simulink model "rugos_rendszer_new"  (R2019b)
settings: Solver=ode23  StartTime=0  StopTime=5  MaxStep=0.1  RelTol=1e-3  AbsTol=1e-6
PostLoadFcn:
  | crtanim2([],[],[],0,1);
model workspace (MAT data in the model file):
  K = [3.08189689488 2.48269889228 0.0803807652926 3.18658131281]
  ae = [0  1  -31.4507297013  0; -1  0  44.8536687603  0; 0  0  -46.6599405981  1; 1  0  -89.5750283103  0]
  be = [0  31.4507297013; 1  -43.8536687603; 0  46.6599405981; 0  88.5750283103]
  ce = [1  0  0  0; 0  1  0  0; 0  0  1  0; 0  0  0  1]
  de = [0  0; 0  0; 0  0; 0  0]
  ka = 1
  m1 = 1
  m2 = 1
  xBx1 = [0; 0; -2; -2; 0]
  xBx2 = [0; 2; 2; 0; 0]
  xSpr = [0; 0.4; 0.8; 1.6; 2.4; 3.2; 3.6; 4]
values from neighbouring files (symbols this model uses):
  k = 2    [Untitled.m]
  Kfb = -inv(R)*B'*P    [Untitled.m]
  Kff = -inv(R)*B'*((A-B*inv(R)*B'*P)')^(-1)*C'*Q    [Untitled.m]
  M1 = 50    [Untitled.m]
  M2 = 10    [Untitled.m]
Description:
  | Double Spring Mass System
  | 
  | This example shows how to model a double spring-mass-damper system with a periodically
  | varying forcing function.  Associated with the example is an animation function
  | that will automatically open a figure window and display to it. In this system,
  | the only sensor is attached to the mass on the left, and the actuator is
  | attached to the mass on the left. State estimation and LQR control are used.
settings Model: ExtModeAutoUpdateStatusClock=off  Creator=The MathWorks, Inc.  LastModifiedBy=patti
settings SolverCC: AutoScaleAbsTol=off
settings DataIOCC: ExternalInput=[]  InitialState=[]  SaveFormat=Array  SaveOutput=off  SaveTime=off  ReturnWorkspaceOutputs=off
settings OptimizationCC: BlockReduction=off  BooleanDataType=off  InitFltsAndDblsToZero=on  LifeSpan=inf  BufferReusableBoundary=off
settings DebuggingCC: SaveWithParameterizedLinksMsg=none  UnderspecifiedInitializationDetection=Classic  MergeDetectMultiDrivingBlocksExec=none  SignalResolutionControl=TryResolveAllWithWarning  MultiTaskDSMMsg=warning  MultiTaskCondExecSysMsg=none  FcnCallInpInsideContextMsg=warning  BusObjectLabelMismatch=none  SFUnexpectedBacktrackingDiag=warning  SFNoUnconditionalDefaultTransitionDiag=warning  SFExecutionAtInitializationDiag=none  ArithmeticOperatorsInVariantConditions=warning
settings HardwareCC: ProdBitPerPointer=32  ProdBitPerSizeT=32  ProdBitPerPtrDiffT=32  ProdLargestAtomicFloat=None  ProdIntDivRoundTo=Undefined  ProdEndianess=Unspecified  ProdWordSize=32  ProdHWDeviceType=32-bit Generic  TargetUnknown=on
settings ModelReferenceCC: PropagateSignalLabelsOutOfModel=off
settings SFSimCC: SimUseLocalCustomCode=off  CustomCodeUndefinedFunction=UseInterfaceOnly
settings RTWCC: Description=Generic Real-Time Target  RTWUseLocalCustomCode=off
settings CodeAppCC: StateflowObjectComments=on
settings GRTTargetCC: TargetFcnLib=ansi_tfl_tmw.mat  TargetLangStandard=C89/C90 (ANSI)  GeneratePreprocessorConditionals=Disable all  CombineOutputUpdateFcns=off  GRTInterface=on
settings ConfigComp: CovMetricSettings=dw  CovHtmlReporting=on  CovSaveCumulativeToWorkspaceVar=on  CovSaveSingleToWorkspaceVar=on  CovExternalEMLEnable=off

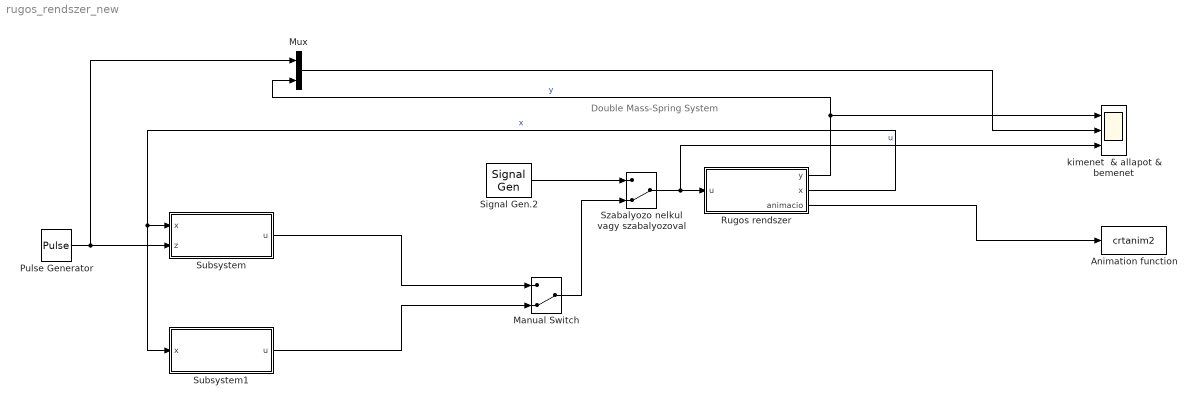
== system rugos_rendszer_new ==
  note: Double Mass-Spring System
  Animation function : S-Function  FunctionName=crtanim2  Parameters=0.1  SFunctionDeploymentMode=off  EnableBusSupport=off
      settings: DeleteFcn=shh = get(0,'ShowHiddenHandles');set(0,'ShowHiddenHandles','on');if ~isempty(findobj('type','figure','name','dblcart1 Animation'));close('dblcart1 Animation'); end;set(0,'ShowHiddenHandles',shh);
  Manual Switch : ManualSwitch  CurrentSetting=0
  Mux : Mux  Inputs=2
  Pulse Generator : DiscretePulseGenerator  PulseType=Time based  Amplitude=5  Period=20  PulseWidth=50
  Rugos rendszer : Subsystem  mask{ka=k, m1=M1, m2=M2}
  Signal Gen.2 : SignalGenerator  WaveForm=square  Amplitude=15  Frequency=0.300000  Units=rad/sec
  Subsystem : Subsystem
  Subsystem1 : Subsystem
  Szabalyozo nelkul vagy szabalyozoval : ManualSwitch  CurrentSetting=0
  kimenet  & allapot & bemenet : Scope  NumInputPorts=3
  wires:
  Signal Gen.2/1 -> Szabalyozo nelkul vagy szabalyozoval/1
  Rugos rendszer/3(animacio) -> Animation function/1
  Szabalyozo nelkul vagy szabalyozoval/1 -> kimenet  & allapot & bemenet/3, Rugos rendszer/1(u)  "u"
  Rugos rendszer/2(x) -> Subsystem1/1("x "), Subsystem/1(x)  "x"
  Manual Switch/1 -> Szabalyozo nelkul vagy szabalyozoval/2
  Subsystem/1("u ") -> Manual Switch/1
  Subsystem1/1("u ") -> Manual Switch/2
  Pulse Generator/1 -> Subsystem/2(z), Mux/1
  Rugos rendszer/1(y) -> kimenet  & allapot & bemenet/1, Mux/2  "y"
  Mux/1 -> kimenet  & allapot & bemenet/2

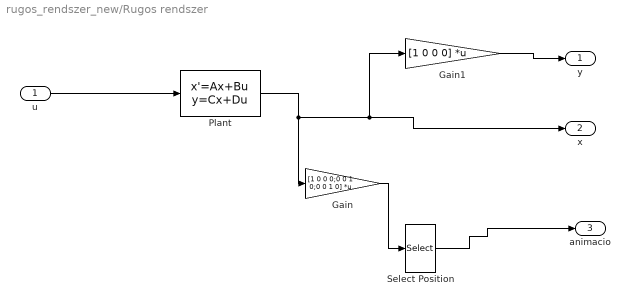
== system rugos_rendszer_new/Rugos rendszer ==
  u : Inport
  Gain : Gain  Gain=[1 0 0 0;0 0 1 0;0 0 1 0]  Multiplication=Matrix(K*u)
  Gain1 : Gain  Gain=[1 0 0 0]  Multiplication=Matrix(K*u)
  Plant : StateSpace  A=[0 1 0 0; -ka/m1 0 ka/m1 0; 0 0 0 1;ka/m2 0 -ka/m2 0]  B=[0; 1; 0; 0]  C=eye(4)  D=zeros(4,1)  InitialCondition=0
  Select Position : Selector  InputPortWidth=3  IndexOptions=Index vector (dialog)  Indices=[1,2]  OutputSizes=1
  y : Outport
  x : Outport  Port=2
  animacio : Outport  Port=3
  wires:
  Select Position/1 -> animacio/1
  u/1 -> Plant/1
  Gain1/1 -> y/1
  Gain/1 -> Select Position/1
  Plant/1 -> Gain1/1, x/1, Gain/1

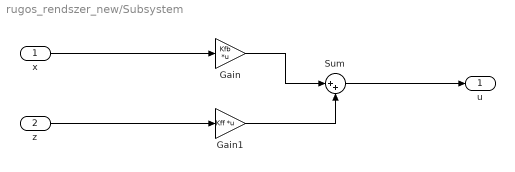
== system rugos_rendszer_new/Subsystem ==
  x : Inport
  z : Inport  Port=2
  Gain : Gain  Gain=Kfb  Multiplication=Matrix(K*u)
  Gain1 : Gain  Gain=Kff  Multiplication=Matrix(K*u)
  Sum : Sum  Inputs=|++
  "u " : Outport
  wires:
  x/1 -> Gain/1
  z/1 -> Gain1/1
  Gain1/1 -> Sum/2
  Gain/1 -> Sum/1
  Sum/1 -> "u "/1

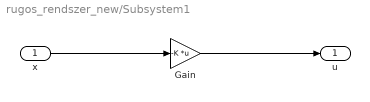
== system rugos_rendszer_new/Subsystem1 ==
  "x " : Inport
  Gain : Gain  Gain=-K  Multiplication=Matrix(K*u)
  "u " : Outport
  wires:
  "x "/1 -> Gain/1
  Gain/1 -> "u "/1
